simulink model "main"  (R2020b)
settings: Solver=VariableStepAuto  StartTime=0.0  StopTime=100.0  RelTol=1e-3
libraries: sharedtransform x1
settings Model: Creator=Dogukan  LastModifiedBy=Dogukan

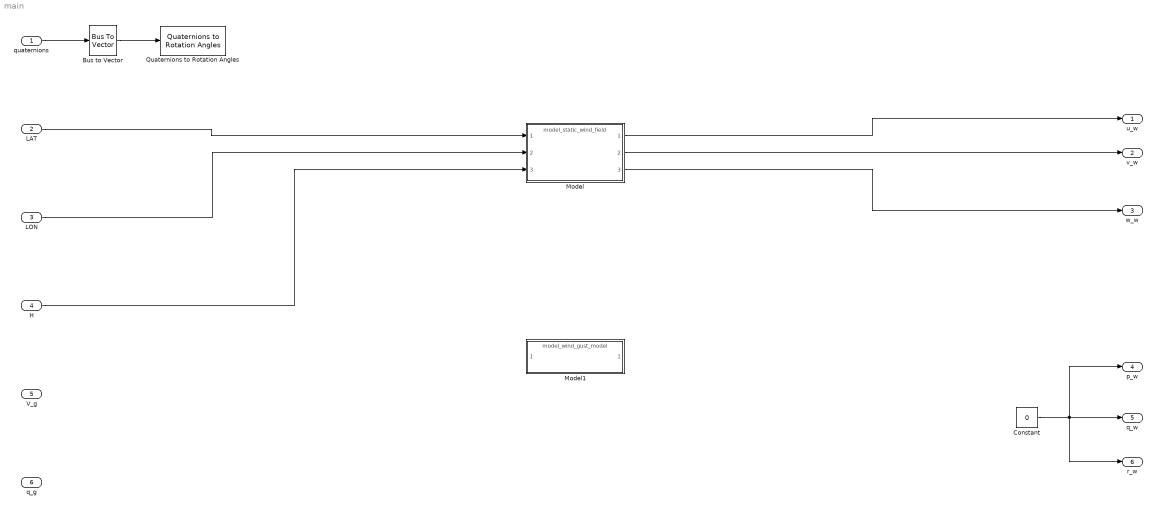
== system main ==
  quaternions : Inport  OutDataTypeStr=Bus: quaternionBus
  LAT : Inport  Port=2
  LON : Inport  Port=3
  H : Inport  Port=4
  V_g : Inport  Port=5  OutDataTypeStr=Bus: velocityBus
  q_g : Inport  Port=6  OutDataTypeStr=Bus: rotationBus
  Bus to Vector : BusToVector
  Constant : Constant  Value=0
  Model : ModelReference  ModelNameDialog=model_static_wind_field.slx  SimulationMode=Normal  ModelReferenceVersion=1.14
  Model1 : ModelReference  ModelNameDialog=model_wind_gust_model.slx  SimulationMode=Normal  ModelReferenceVersion=1.1
  Quaternions to Rotation Angles : sharedtransform/Quaternions to Rotation Angles  rotationOrder=ZYX  aMode=aMode
      settings: SourceProductBaseCode=AE,PW,MT,UV,VE,VP
  u_w : Outport  SignalName=u_w  OutDataTypeStr=double
  v_w : Outport  Port=2  SignalName=v_w  OutDataTypeStr=double
  w_w : Outport  Port=3  SignalName=w_w  OutDataTypeStr=double
  p_w : Outport  Port=4  SignalName=p_w  OutDataTypeStr=double
  q_w : Outport  Port=5  SignalName=q_w  OutDataTypeStr=double
  r_w : Outport  Port=6  SignalName=r_w  OutDataTypeStr=double
  wires:
  LAT/1 -> Model/1
  LON/1 -> Model/2
  H/1 -> Model/3
  Constant/1 -> q_w/1, p_w/1, r_w/1
  quaternions/1 -> Bus to Vector/1
  Bus to Vector/1 -> Quaternions to Rotation Angles/1
  Model/1 -> u_w/1
  Model/2 -> v_w/1
  Model/3 -> w_w/1
